simulink model "HW1"  (R2019b)
settings: Solver=VariableStepAuto  StartTime=0.0  StopTime=10  RelTol=1e-3
settings Model: Creator=mason  LastModifiedBy=mason

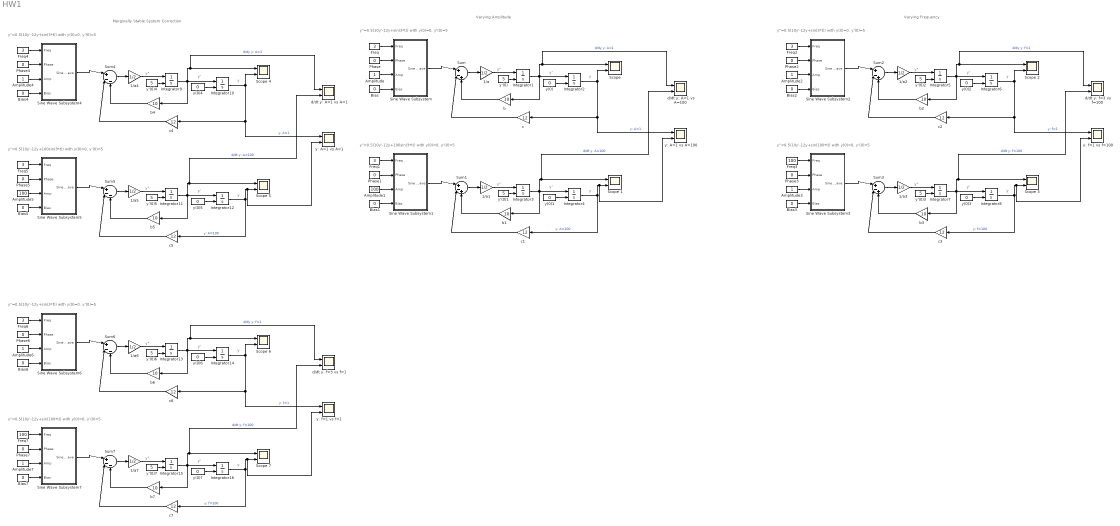
== system HW1 ==
  note: Varying Amplitude
  note: y"
  note: y
  note: y'
  note: y"=0.5(10y'-12y+sin(3*t))
      | with y(0)=0, y'(0)=5
  note: y"=0.5(10y'-12y+100sin(3*t))
      | with y(0)=0, y'(0)=5
  note: y"
  note: y
  note: y'
  note: y"=0.5(10y'-12y+sin(3*t))
      | with y(0)=0, y'(0)=5
  note: y'
  note: y"
  note: y
  note: y"
  note: y"=0.5(10y'-12y+sin(100*t))
      | with y(0)=0, y'(0)=5
  note: y'
  note: y
  note: Varying Frequency
  note: Marginally Stable System Correction
  note: y"=0.5(10y'-12y+sin(3*t))
      | with y(0)=0, y'(0)=5
  note: y'
  note: y"
  note: y
  note: y"
  note: y"=0.5(10y'-12y+100sin(3*t))
      | with y(0)=0, y'(0)=5
  note: y'
  note: y
  note: y
  note: y"=0.5(10y'-12y+sin(3*t))
      | with y(0)=0, y'(0)=5
  note: y'
  note: y"
  note: y
  note: y'
  note: y"
  note: y"=0.5(10y'-12y+sin(100*t))
      | with y(0)=0, y'(0)=5
  " d/dt y: A=1 vs A=1" : Scope  NumInputPorts=2
  " d/dt y: A=1 vs A=100" : Scope  NumInputPorts=2
  " d/dt y: f=3 vs f=1" : Scope  NumInputPorts=2
  " d/dt y: f=3 vs f=100" : Scope  NumInputPorts=2
  " y: A=1 vs A=1" : Scope  NumInputPorts=2
  " y: A=1 vs A=100" : Scope  NumInputPorts=2
  " y: f=1 vs f=1" : Scope  NumInputPorts=2
  " y: f=1 vs f=100" : Scope  NumInputPorts=2
  1/a{,1..7} (8 alike) : Gain  Gain=1/2
  Amplitude{,2..4,6..7} (6 alike) : Constant
  Amplitude1 : Constant  Value=100
  Amplitude5 : Constant  Value=100
  Bias{,1..7} (8 alike) : Constant  Value=0
  Freq{,1..2,4..6} (6 alike) : Constant  Value=3
  Freq3 : Constant  Value=100
  Freq7 : Constant  Value=100
  Integrator{1..16} (16 alike) : Integrator  InitialConditionSource=external
  Phase{,1..7} (8 alike) : Constant  Value=0
  Scope {,1..7} (8 alike) : Scope  NumInputPorts=2
  Sine Wave Subsystem : Subsystem
  Sine Wave Subsystem1 : Subsystem
  Sine Wave Subsystem2 : Subsystem
  Sine Wave Subsystem3 : Subsystem
  Sine Wave Subsystem4 : Subsystem
  Sine Wave Subsystem5 : Subsystem
  Sine Wave Subsystem6 : Subsystem
  Sine Wave Subsystem7 : Subsystem
  Sum{,1..3} (4 alike) : Sum  Inputs=|+-+
  Sum{4..7} (4 alike) : Sum  Inputs=|+--
  b{,1..7} (8 alike) : Gain  Gain=10
  c{,1..7} (8 alike) : Gain  Gain=12
  y'(0){,1..7} (8 alike) : Constant  Value=5
  y(0){,1..7} (8 alike) : Constant  Value=0
  wires:
  1/a/1 -> Integrator1/1
  y(0)/1 -> Integrator2/2
  c/1 -> Sum/2
  Sum/1 -> 1/a/1
  b/1 -> Sum/3
  y'(0)/1 -> Integrator1/2
  Integrator1/1 -> " d/dt y: A=1 vs A=100"/1, "Scope "/1, Integrator2/1, b/1  "d/dy y: A=1"
  Integrator2/1 -> " y: A=1 vs A=100"/1, c/1, "Scope "/2  "y: A=1"
  Freq/1 -> Sine Wave Subsystem/1(Freq)
  Phase/1 -> Sine Wave Subsystem/2(Phase)
  Amplitude/1 -> Sine Wave Subsystem/3(Amp)
  Bias/1 -> Sine Wave Subsystem/4(Bias)
  Sine Wave Subsystem/1(Sine Wave) -> Sum/1
  Bias1/1 -> Sine Wave Subsystem1/4(Bias)
  Phase1/1 -> Sine Wave Subsystem1/2(Phase)
  Integrator4/1 -> " y: A=1 vs A=100"/2, Scope 1/2, c1/1  "y: A=100"
  c1/1 -> Sum1/2
  Sine Wave Subsystem1/1(Sine Wave) -> Sum1/1
  y'(0)1/1 -> Integrator3/2
  Sum1/1 -> 1/a1/1
  Integrator3/1 -> " d/dt y: A=1 vs A=100"/2, Scope 1/1, Integrator4/1, b1/1  "d/dt y: A=100"
  Freq1/1 -> Sine Wave Subsystem1/1(Freq)
  Amplitude1/1 -> Sine Wave Subsystem1/3(Amp)
  y(0)1/1 -> Integrator4/2
  1/a1/1 -> Integrator3/1
  b1/1 -> Sum1/3
  Phase2/1 -> Sine Wave Subsystem2/2(Phase)
  1/a3/1 -> Integrator7/1
  b3/1 -> Sum3/3
  Freq3/1 -> Sine Wave Subsystem3/1(Freq)
  Amplitude3/1 -> Sine Wave Subsystem3/3(Amp)
  y(0)3/1 -> Integrator8/2
  Phase3/1 -> Sine Wave Subsystem3/2(Phase)
  Sine Wave Subsystem3/1(Sine Wave) -> Sum3/1
  Sum3/1 -> 1/a3/1
  Bias3/1 -> Sine Wave Subsystem3/4(Bias)
  c3/1 -> Sum3/2
  Integrator6/1 -> " y: f=1 vs f=100"/1, c2/1, Scope 2/2  "y: f=1"
  y'(0)3/1 -> Integrator7/2
  Integrator5/1 -> " d/dt y: f=3 vs f=100"/1, Scope 2/1, Integrator6/1, b2/1  "d/dy y: f=1"
  Freq2/1 -> Sine Wave Subsystem2/1(Freq)
  Amplitude2/1 -> Sine Wave Subsystem2/3(Amp)
  c2/1 -> Sum2/2
  Integrator8/1 -> " y: f=1 vs f=100"/2, Scope 3/2, c3/1  "y: f=100"
  Integrator7/1 -> " d/dt y: f=3 vs f=100"/2, Scope 3/1, Integrator8/1, b3/1  "d/dt y: f=100"
  Sine Wave Subsystem2/1(Sine Wave) -> Sum2/1
  b2/1 -> Sum2/3
  y'(0)2/1 -> Integrator5/2
  y(0)2/1 -> Integrator6/2
  1/a2/1 -> Integrator5/1
  Bias2/1 -> Sine Wave Subsystem2/4(Bias)
  Sum2/1 -> 1/a2/1
  Phase4/1 -> Sine Wave Subsystem4/2(Phase)
  1/a5/1 -> Integrator11/1
  b5/1 -> Sum5/3
  Freq5/1 -> Sine Wave Subsystem5/1(Freq)
  Amplitude5/1 -> Sine Wave Subsystem5/3(Amp)
  y(0)5/1 -> Integrator12/2
  Phase5/1 -> Sine Wave Subsystem5/2(Phase)
  Sine Wave Subsystem5/1(Sine Wave) -> Sum5/1
  Sum5/1 -> 1/a5/1
  Bias5/1 -> Sine Wave Subsystem5/4(Bias)
  c5/1 -> Sum5/2
  Integrator10/1 -> " y: A=1 vs A=1"/1, c4/1, Scope 4/2  "y: A=1"
  y'(0)5/1 -> Integrator11/2
  Integrator9/1 -> " d/dt y: A=1 vs A=1"/1, Scope 4/1, Integrator10/1, b4/1  "d/dy y: A=1"
  Freq4/1 -> Sine Wave Subsystem4/1(Freq)
  Amplitude4/1 -> Sine Wave Subsystem4/3(Amp)
  c4/1 -> Sum4/2
  Integrator12/1 -> " y: A=1 vs A=1"/2, Scope 5/2, c5/1  "y: A=100"
  Integrator11/1 -> " d/dt y: A=1 vs A=1"/2, Scope 5/1, Integrator12/1, b5/1  "d/dt y: A=100"
  Sine Wave Subsystem4/1(Sine Wave) -> Sum4/1
  b4/1 -> Sum4/3
  y'(0)4/1 -> Integrator9/2
  y(0)4/1 -> Integrator10/2
  1/a4/1 -> Integrator9/1
  Bias4/1 -> Sine Wave Subsystem4/4(Bias)
  Sum4/1 -> 1/a4/1
  y(0)6/1 -> Integrator14/2
  Bias6/1 -> Sine Wave Subsystem6/4(Bias)
  1/a6/1 -> Integrator13/1
  y'(0)6/1 -> Integrator13/2
  b6/1 -> Sum6/3
  Sine Wave Subsystem6/1(Sine Wave) -> Sum6/1
  1/a7/1 -> Integrator15/1
  Integrator15/1 -> " d/dt y: f=3 vs f=1"/2, Scope 7/1, Integrator16/1, b7/1  "d/dt y: f=100"
  Amplitude7/1 -> Sine Wave Subsystem7/3(Amp)
  Phase6/1 -> Sine Wave Subsystem6/2(Phase)
  Bias7/1 -> Sine Wave Subsystem7/4(Bias)
  Sum7/1 -> 1/a7/1
  Sine Wave Subsystem7/1(Sine Wave) -> Sum7/1
  Phase7/1 -> Sine Wave Subsystem7/2(Phase)
  y(0)7/1 -> Integrator16/2
  c6/1 -> Sum6/2
  Amplitude6/1 -> Sine Wave Subsystem6/3(Amp)
  Freq6/1 -> Sine Wave Subsystem6/1(Freq)
  c7/1 -> Sum7/2
  Integrator14/1 -> " y: f=1 vs f=1"/1, c6/1, Scope 6/2  "y: f=1"
  b7/1 -> Sum7/3
  y'(0)7/1 -> Integrator15/2
  Sum6/1 -> 1/a6/1
  Integrator13/1 -> " d/dt y: f=3 vs f=1"/1, Scope 6/1, Integrator14/1, b6/1  "d/dy y: f=1"
  Freq7/1 -> Sine Wave Subsystem7/1(Freq)
  Integrator16/1 -> " y: f=1 vs f=1"/2, Scope 7/2, c7/1  "y: f=100"

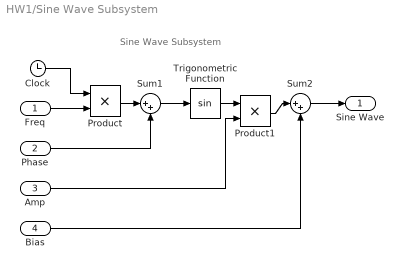
== system HW1/Sine Wave Subsystem ==
  note: Sine Wave Subsystem
  Freq : Inport
  Phase : Inport  Port=2
  Amp : Inport  Port=3
  Bias : Inport  Port=4
  Clock : Clock
  Product : Product
  Product1 : Product
  Sum1 : Sum  Inputs=|++
  Sum2 : Sum  Inputs=|++
  Trigonometric Function : Trigonometry
  Sine Wave : Outport
  wires:
  Trigonometric Function/1 -> Product1/1
  Freq/1 -> Product/2
  Clock/1 -> Product/1
  Phase/1 -> Sum1/2
  Product1/1 -> Sum2/1
  Product/1 -> Sum1/1
  Amp/1 -> Product1/2
  Bias/1 -> Sum2/2
  Sum1/1 -> Trigonometric Function/1
  Sum2/1 -> Sine Wave/1

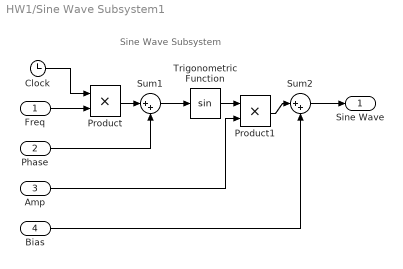
== system HW1/Sine Wave Subsystem1 ==
  note: Sine Wave Subsystem
  Freq : Inport
  Phase : Inport  Port=2
  Amp : Inport  Port=3
  Bias : Inport  Port=4
  Clock : Clock
  Product : Product
  Product1 : Product
  Sum1 : Sum  Inputs=|++
  Sum2 : Sum  Inputs=|++
  Trigonometric Function : Trigonometry
  Sine Wave : Outport
  wires:
  Trigonometric Function/1 -> Product1/1
  Freq/1 -> Product/2
  Clock/1 -> Product/1
  Phase/1 -> Sum1/2
  Product1/1 -> Sum2/1
  Product/1 -> Sum1/1
  Amp/1 -> Product1/2
  Bias/1 -> Sum2/2
  Sum1/1 -> Trigonometric Function/1
  Sum2/1 -> Sine Wave/1

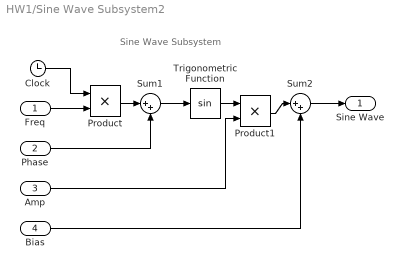
== system HW1/Sine Wave Subsystem2 ==
  note: Sine Wave Subsystem
  Freq : Inport
  Phase : Inport  Port=2
  Amp : Inport  Port=3
  Bias : Inport  Port=4
  Clock : Clock
  Product : Product
  Product1 : Product
  Sum1 : Sum  Inputs=|++
  Sum2 : Sum  Inputs=|++
  Trigonometric Function : Trigonometry
  Sine Wave : Outport
  wires:
  Trigonometric Function/1 -> Product1/1
  Freq/1 -> Product/2
  Clock/1 -> Product/1
  Phase/1 -> Sum1/2
  Product1/1 -> Sum2/1
  Product/1 -> Sum1/1
  Amp/1 -> Product1/2
  Bias/1 -> Sum2/2
  Sum1/1 -> Trigonometric Function/1
  Sum2/1 -> Sine Wave/1

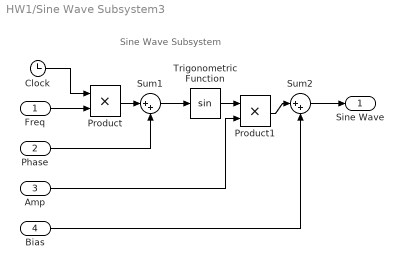
== system HW1/Sine Wave Subsystem3 ==
  note: Sine Wave Subsystem
  Freq : Inport
  Phase : Inport  Port=2
  Amp : Inport  Port=3
  Bias : Inport  Port=4
  Clock : Clock
  Product : Product
  Product1 : Product
  Sum1 : Sum  Inputs=|++
  Sum2 : Sum  Inputs=|++
  Trigonometric Function : Trigonometry
  Sine Wave : Outport
  wires:
  Trigonometric Function/1 -> Product1/1
  Freq/1 -> Product/2
  Clock/1 -> Product/1
  Phase/1 -> Sum1/2
  Product1/1 -> Sum2/1
  Product/1 -> Sum1/1
  Amp/1 -> Product1/2
  Bias/1 -> Sum2/2
  Sum1/1 -> Trigonometric Function/1
  Sum2/1 -> Sine Wave/1

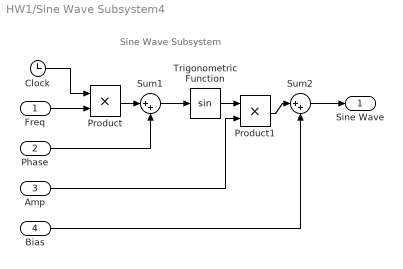
== system HW1/Sine Wave Subsystem4 ==
  note: Sine Wave Subsystem
  Freq : Inport
  Phase : Inport  Port=2
  Amp : Inport  Port=3
  Bias : Inport  Port=4
  Clock : Clock
  Product : Product
  Product1 : Product
  Sum1 : Sum  Inputs=|++
  Sum2 : Sum  Inputs=|++
  Trigonometric Function : Trigonometry
  Sine Wave : Outport
  wires:
  Trigonometric Function/1 -> Product1/1
  Freq/1 -> Product/2
  Clock/1 -> Product/1
  Phase/1 -> Sum1/2
  Product1/1 -> Sum2/1
  Product/1 -> Sum1/1
  Amp/1 -> Product1/2
  Bias/1 -> Sum2/2
  Sum1/1 -> Trigonometric Function/1
  Sum2/1 -> Sine Wave/1

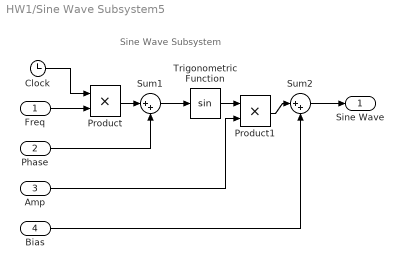
== system HW1/Sine Wave Subsystem5 ==
  note: Sine Wave Subsystem
  Freq : Inport
  Phase : Inport  Port=2
  Amp : Inport  Port=3
  Bias : Inport  Port=4
  Clock : Clock
  Product : Product
  Product1 : Product
  Sum1 : Sum  Inputs=|++
  Sum2 : Sum  Inputs=|++
  Trigonometric Function : Trigonometry
  Sine Wave : Outport
  wires:
  Trigonometric Function/1 -> Product1/1
  Freq/1 -> Product/2
  Clock/1 -> Product/1
  Phase/1 -> Sum1/2
  Product1/1 -> Sum2/1
  Product/1 -> Sum1/1
  Amp/1 -> Product1/2
  Bias/1 -> Sum2/2
  Sum1/1 -> Trigonometric Function/1
  Sum2/1 -> Sine Wave/1

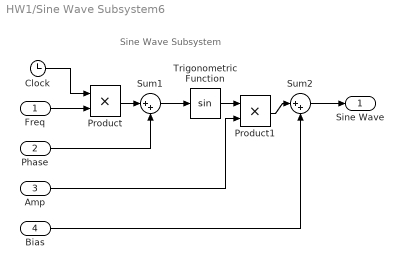
== system HW1/Sine Wave Subsystem6 ==
  note: Sine Wave Subsystem
  Freq : Inport
  Phase : Inport  Port=2
  Amp : Inport  Port=3
  Bias : Inport  Port=4
  Clock : Clock
  Product : Product
  Product1 : Product
  Sum1 : Sum  Inputs=|++
  Sum2 : Sum  Inputs=|++
  Trigonometric Function : Trigonometry
  Sine Wave : Outport
  wires:
  Trigonometric Function/1 -> Product1/1
  Freq/1 -> Product/2
  Clock/1 -> Product/1
  Phase/1 -> Sum1/2
  Product1/1 -> Sum2/1
  Product/1 -> Sum1/1
  Amp/1 -> Product1/2
  Bias/1 -> Sum2/2
  Sum1/1 -> Trigonometric Function/1
  Sum2/1 -> Sine Wave/1

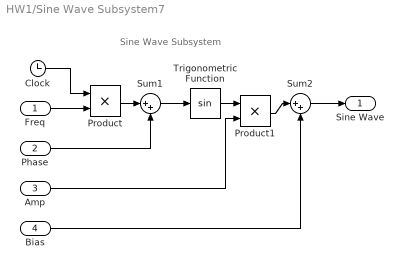
== system HW1/Sine Wave Subsystem7 ==
  note: Sine Wave Subsystem
  Freq : Inport
  Phase : Inport  Port=2
  Amp : Inport  Port=3
  Bias : Inport  Port=4
  Clock : Clock
  Product : Product
  Product1 : Product
  Sum1 : Sum  Inputs=|++
  Sum2 : Sum  Inputs=|++
  Trigonometric Function : Trigonometry
  Sine Wave : Outport
  wires:
  Trigonometric Function/1 -> Product1/1
  Freq/1 -> Product/2
  Clock/1 -> Product/1
  Phase/1 -> Sum1/2
  Product1/1 -> Sum2/1
  Product/1 -> Sum1/1
  Amp/1 -> Product1/2
  Bias/1 -> Sum2/2
  Sum1/1 -> Trigonometric Function/1
  Sum2/1 -> Sine Wave/1
